simulink model "ex1"  (R2023b)
settings: Solver=VariableStepAuto  StartTime=0.0  StopTime=50  RelTol=1e-3
values from neighbouring files (symbols this model uses):
  A = [-1/Ta -ke/La; km/J 0]    [tema6_ts.m]
  B = [kE/La 0; 0 -1/J]    [tema6_ts.m]
  C = [1 0; 0 1]    [tema6_ts.m]
  D = [0 0; 0 0]    [tema6_ts.m]
  J = 0.0302    [tema6_ts.m]
  kE = 42.85    [tema6_ts.m]
  ke = 0.56    [tema6_ts.m]
  kf = 0    [tema6_ts.m]
  km = 0.55    [tema6_ts.m]
  Ra = 5.1    [tema6_ts.m]
  Ta = 0.1    [tema6_ts.m]
  Tm = 0.5    [tema6_ts.m]
settings Model: Creator=chapo  LastModifiedBy=chapo

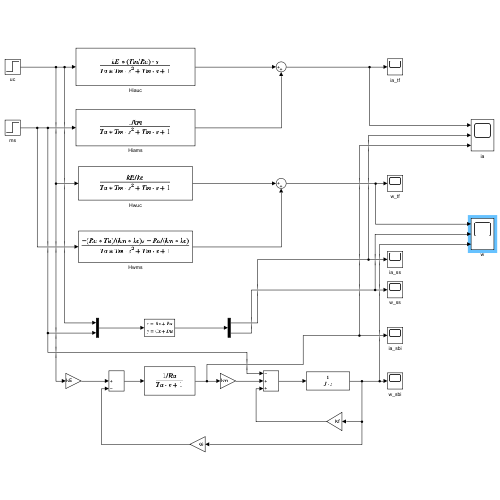
[thumbnail: Simulink's stored preview of the top-level diagram]
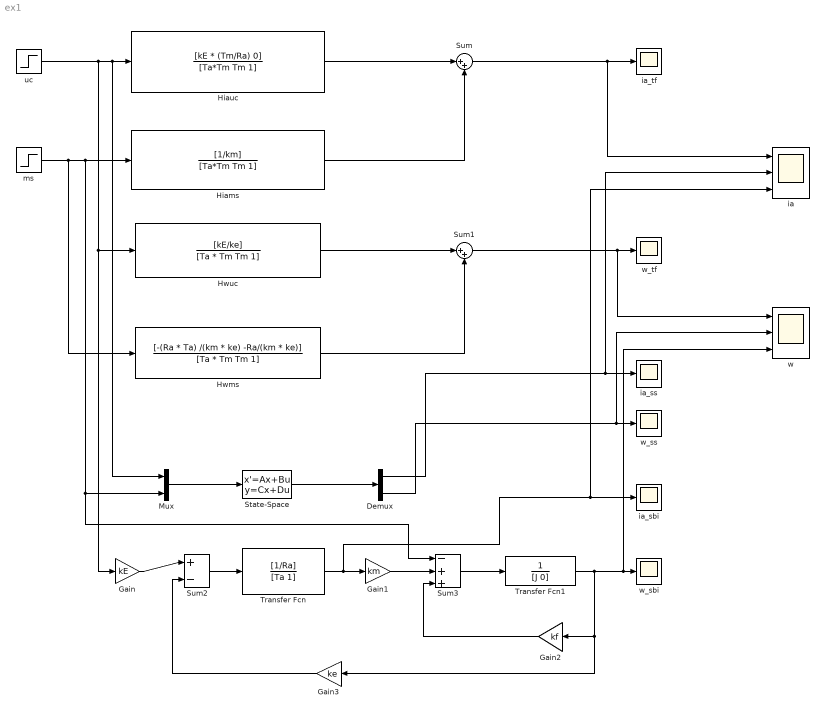
== system ex1 ==
  Demux : Demux  Outputs=2
  Gain : Gain  Gain=kE
  Gain1 : Gain  Gain=km
  Gain2 : Gain  Gain=kf
  Gain3 : Gain  Gain=ke
  Hiams : TransferFcn  Numerator=[1/km]  Denominator=[Ta*Tm Tm 1]
  Hiauc : TransferFcn  Numerator=[kE * (Tm/Ra) 0]  Denominator=[Ta*Tm Tm 1]
  Hwms : TransferFcn  Numerator=[-(Ra * Ta) /(km * ke) -Ra/(km * ke)]  Denominator=[Ta * Tm Tm 1]
  Hwuc : TransferFcn  Numerator=[kE/ke]  Denominator=[Ta * Tm Tm 1]
  Mux : Mux  Inputs=2
  State-Space : StateSpace  A=A  B=B  C=C  D=D  InitialCondition=0
  Sum : Sum  Inputs=|++
  Sum1 : Sum  Inputs=|++
  Sum2 : Sum  Inputs=|+-
  Sum3 : Sum  Inputs=-++
  Transfer Fcn : TransferFcn  Numerator=[1/Ra]  Denominator=[Ta 1]
  Transfer Fcn1 : TransferFcn  Denominator=[J 0]
  ia : Scope  NumInputPorts=3
  ia_sbi : Scope
  ia_ss : Scope
  ia_tf : Scope
  ms : Step  Time=30  SampleTime=0
  uc : Step  Time=0  After=3.5  SampleTime=0
  w : Scope  NumInputPorts=3
  w_sbi : Scope
  w_ss : Scope
  w_tf : Scope
  wires:
  ms/1 -> Hwms/1, Sum3/1, Mux/2, Hiams/1
  uc/1 -> Gain/1, Hwuc/1, Mux/1, Hiauc/1
  Hiauc/1 -> Sum/1
  Hiams/1 -> Sum/2
  Hwuc/1 -> Sum1/1
  Hwms/1 -> Sum1/2
  Sum1/1 -> w/1, w_tf/1
  Sum/1 -> ia/1, ia_tf/1
  Mux/1 -> State-Space/1
  State-Space/1 -> Demux/1
  Demux/2 -> w/2, w_ss/1
  Demux/1 -> ia/2, ia_ss/1
  Sum2/1 -> Transfer Fcn/1
  Gain/1 -> Sum2/1
  Transfer Fcn/1 -> ia/3, ia_sbi/1, Gain1/1
  Gain1/1 -> Sum3/2
  Gain2/1 -> Sum3/3
  Sum3/1 -> Transfer Fcn1/1
  Transfer Fcn1/1 -> Gain3/1, Gain2/1, w/3, w_sbi/1
  Gain3/1 -> Sum2/2
